simulink model "ultrasound"  (Simulink 4.00)
settings: Solver=ode45  StartTime=0.0  StopTime=5  RelTol=1e-3
libraries: truetime x4
settings Model: Creator=anton  LastModifiedBy=anton  UnconnectedInputMsg=none  UnconnectedOutputMsg=none  UnconnectedLineMsg=none  ExtModeAutoUpdateStatusClock=off

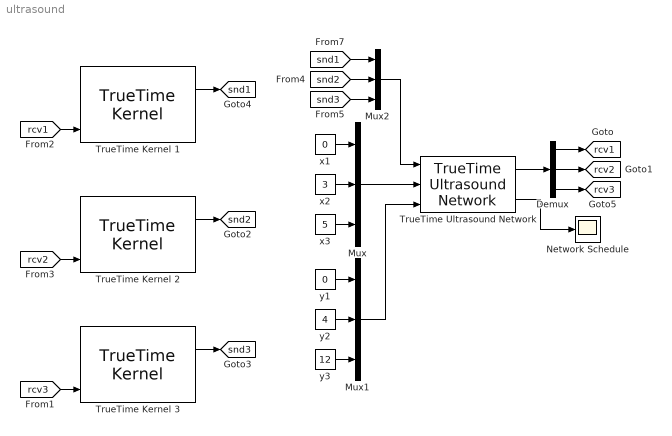
== system ultrasound ==
  Demux : Demux  Outputs=3  BusSelectionMode=off
  Mux : Mux  Inputs=3
  Mux1 : Mux  Inputs=3
  Mux2 : Mux  Inputs=3
  Network Schedule : Scope
      settings: TimeRange=10  YMin=1  YMax=2.5  SaveName=nschedule  MaxDataPoints=5000
  TrueTime Kernel 1 : truetime/TrueTime Kernel  sfun=node_init  args=1  battery=off  clockdrift=0  clockoffset=0
  TrueTime Kernel 2 : truetime/TrueTime Kernel  sfun=node_init  args=2  battery=off  clockdrift=0  clockoffset=0
  TrueTime Kernel 3 : truetime/TrueTime Kernel  sfun=node_init  args=3  battery=off  clockdrift=0  clockoffset=0
  TrueTime Ultrasound Network : truetime/TrueTime Ultrasound Network  AncestorBlock="truetime/TrueTime Wireless  Network"  nwnbr=1  nnodes=3  reach=10  pinglength=0.001  speedofsound=344
  x1 : Constant  Value=0
  x2 : Constant  Value=3
  x3 : Constant  Value=5
  y1 : Constant  Value=0
  y2 : Constant  Value=4
  y3 : Constant  Value=12
  tag scope: rcv1=global, rcv2=global, rcv3=global, snd1=global, snd2=global, snd3=global
  wires:
  x1/1 -> Mux/1
  y1/1 -> Mux1/1
  x2/1 -> Mux/2
  y2/1 -> Mux1/2
  Mux/1 -> TrueTime Ultrasound Network/2
  Mux1/1 -> TrueTime Ultrasound Network/3
  TrueTime Ultrasound Network/2 -> Network Schedule/1
  [snd1] -> Mux2/1
  [snd2] -> Mux2/2
  Mux2/1 -> TrueTime Ultrasound Network/1
  TrueTime Ultrasound Network/1 -> Demux/1
  Demux/1 -> [rcv1]
  Demux/2 -> [rcv2]
  TrueTime Kernel 1/2 -> [snd1]
  TrueTime Kernel 2/2 -> [snd2]
  [rcv1] -> TrueTime Kernel 1/3
  [rcv2] -> TrueTime Kernel 2/3
  TrueTime Kernel 3/2 -> [snd3]
  [rcv3] -> TrueTime Kernel 3/3
  x3/1 -> Mux/3
  y3/1 -> Mux1/3
  [snd3] -> Mux2/3
  Demux/3 -> [rcv3]
